simulink model "heater_switch_Template"  (R2021a)
settings: Solver=VariableStepAuto  StartTime=0.0  StopTime=10.0  RelTol=1e-3
settings Model: Creator=Intuito_PC  LastModifiedBy=Intuito_PC

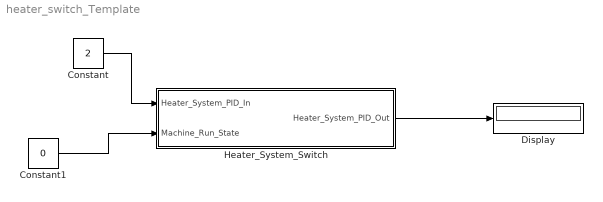
== system heater_switch_Template ==
  Constant : Constant  Value=2
  Constant1 : Constant  Value=0
  Display : Display
  Heater_System_Switch : MATLAB Function  TreatAsAtomicUnit=on
  wires:
  Heater_System_Switch/1(Heater_System_PID_Out) -> Display/1
  Constant/1 -> Heater_System_Switch/1(Heater_System_PID_In)
  Constant1/1 -> Heater_System_Switch/2(Machine_Run_State)

== matlab function heater_switch_Template/Heater_System_Switch ==
  data: Heater_System_PID_In input; Heater_System_PID_Out output; Machine_Run_State input
function Heater_System_PID_Out = fcn(Heater_System_PID_In, Machine_Run_State)
% Check Machine Run State
if Machine_Run_State == 1  % “Standby”, “Running” : (0, 1)
    Heater_System_PID_Out = Heater_System_PID_In; % ON Value
else 
    Heater_System_PID_Out = 0; % OFF Value
end
